simulink model "motion_joints"  (R2020a)
settings: Solver=ode1  StartTime=0.0  StopTime=10  FixedStep=0.001  RelTol=1e-3
libraries: robotcorelib x2, robotmaniplib x2
settings Model: Creator=Robot  LastModifiedBy=Robot

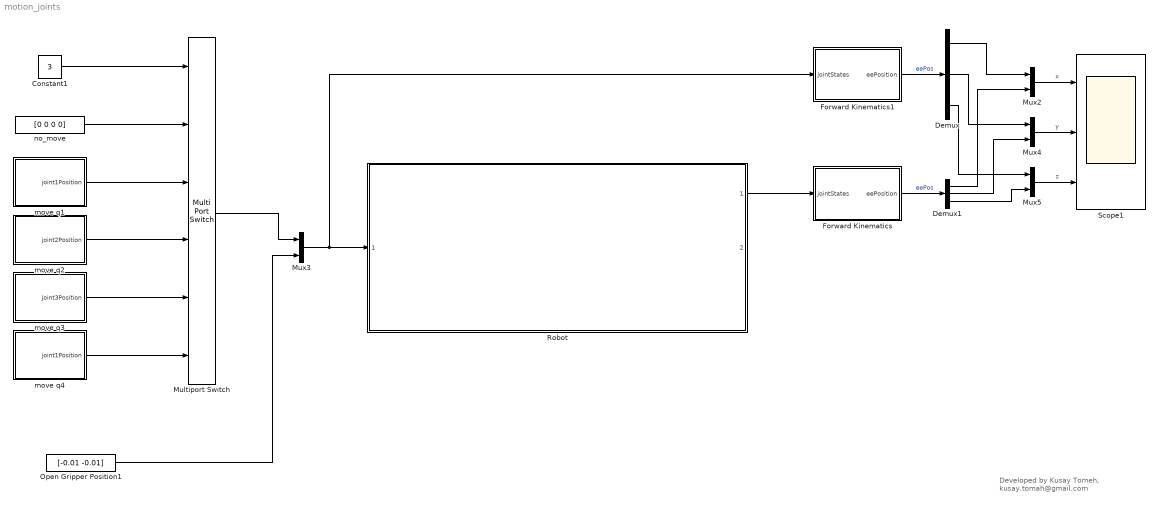
== system motion_joints ==
  note: Developed by Kusay Tomeh,
      | kusay.tomah@gmail.com
  Constant1 : Constant  Value=3
  Demux : Demux  Outputs=3
  Demux1 : Demux  Outputs=3
  Forward Kinematics : Subsystem
  Forward Kinematics1 : Subsystem
  Multiport Switch : MultiPortSwitch  Inputs=5
  Mux{2..5} (4 alike) : Mux  Inputs=2
  Open Gripper Position1 : Constant  Value=[-0.01 -0.01]
  Robot : Subsystem  ReferencedSubsystem=RobotModelWithFloor
  Scope1 : Scope  NumInputPorts=3
  move q1 : Subsystem
  move q2 : Subsystem
  move q3 : Subsystem
  move q4 : Subsystem
  no_move : Constant  Value=[0 0 0 0]
  wires:
  Mux3/1 -> Forward Kinematics1/1(jointStates), Robot/1
  Open Gripper Position1/1 -> Mux3/2
  move q4/1(joint1Position) -> Multiport Switch/6
  move q3/1(joint3Position) -> Multiport Switch/5
  move q2/1(joint2Position) -> Multiport Switch/4
  move q1/1(joint1Position) -> Multiport Switch/3
  Constant1/1 -> Multiport Switch/1
  Mux2/1 -> Scope1/1  "x"
  Multiport Switch/1 -> Mux3/1
  Demux1/2 -> Mux4/2
  Mux4/1 -> Scope1/2  "y"
  Demux/1 -> Mux2/1
  Demux/3 -> Mux5/1
  Demux1/3 -> Mux5/2
  Robot/1 -> Forward Kinematics/1(jointStates)
  Demux/2 -> Mux4/1
  Mux5/1 -> Scope1/3  "z"
  Demux1/1 -> Mux2/2
  Forward Kinematics/1(eePosition) -> Demux1/1  "eePos"
  Forward Kinematics1/1(eePosition) -> Demux/1  "eePos"
  no_move/1 -> Multiport Switch/2

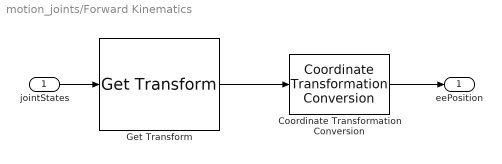
== system motion_joints/Forward Kinematics ==
  jointStates : Inport
  Coordinate Transformation Conversion : robotcorelib/Coordinate Transformation Conversion  InputRepresentation=Homogeneous Transformation  InputEulerSequence=ZYX  ShowTrVecInputPort=on  OutputRepresentation=Translation Vector  OutputEulerSequence=ZYX  ShowTrVecOutputPort=on  SimulateUsing=Code generation
      settings: SourceProductBaseCode=NV,RO,RR
      settings: AttributesFormatString=|
      | %<InputRepresentation>
      | to %<OutputRepresentation>
  Get Transform : robotmaniplib/Get Transform  RigidBodyTree=robot  SourceBody=end_effector  TargetBody=world  SimulateUsing=Interpreted execution
  eePosition : Outport  VectorParamsAs1DForOutWhenUnconnected=off
  wires:
  jointStates/1 -> Get Transform/1
  Coordinate Transformation Conversion/1 -> eePosition/1
  Get Transform/1 -> Coordinate Transformation Conversion/1

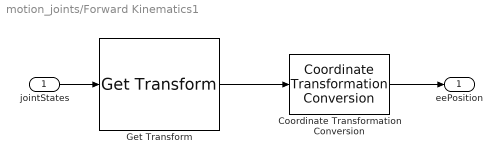
== system motion_joints/Forward Kinematics1 ==
  jointStates : Inport
  Coordinate Transformation Conversion : robotcorelib/Coordinate Transformation Conversion  InputRepresentation=Homogeneous Transformation  InputEulerSequence=ZYX  ShowTrVecInputPort=on  OutputRepresentation=Translation Vector  OutputEulerSequence=ZYX  ShowTrVecOutputPort=on  SimulateUsing=Code generation
      settings: SourceProductBaseCode=NV,RO,RR
      settings: AttributesFormatString=|
      | %<InputRepresentation>
      | to %<OutputRepresentation>
  Get Transform : robotmaniplib/Get Transform  RigidBodyTree=robot  SourceBody=end_effector  TargetBody=world  SimulateUsing=Interpreted execution
  eePosition : Outport  VectorParamsAs1DForOutWhenUnconnected=off
  wires:
  Get Transform/1 -> Coordinate Transformation Conversion/1
  Coordinate Transformation Conversion/1 -> eePosition/1
  jointStates/1 -> Get Transform/1

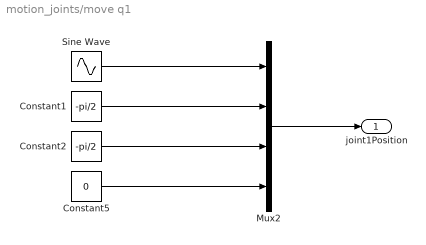
== system motion_joints/move q1 ==
  Constant1 : Constant  Value=-pi/2
  Constant2 : Constant  Value=-pi/2
  Constant5 : Constant  Value=0
  Mux2 : Mux
  Sine Wave : Sin  Amplitude=3.14  SampleTime=0
  joint1Position : Outport
  wires:
  Constant5/1 -> Mux2/4
  Constant2/1 -> Mux2/3
  Mux2/1 -> joint1Position/1
  Sine Wave/1 -> Mux2/1
  Constant1/1 -> Mux2/2

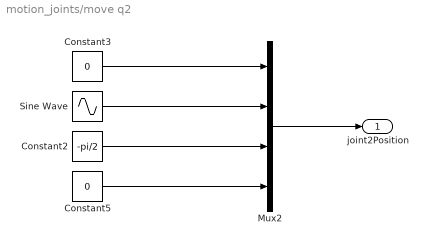
== system motion_joints/move q2 ==
  Constant2 : Constant  Value=-pi/2
  Constant3 : Constant  Value=0
  Constant5 : Constant  Value=0
  Mux2 : Mux
  Sine Wave : Sin  Amplitude=pi/2  SampleTime=0
  joint2Position : Outport
  wires:
  Sine Wave/1 -> Mux2/2
  Constant3/1 -> Mux2/1
  Mux2/1 -> joint2Position/1
  Constant2/1 -> Mux2/3
  Constant5/1 -> Mux2/4

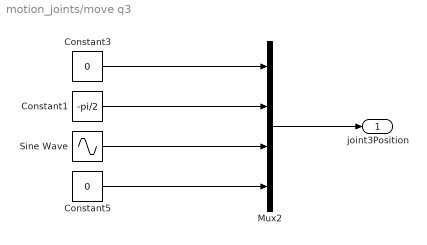
== system motion_joints/move q3 ==
  Constant1 : Constant  Value=-pi/2
  Constant3 : Constant  Value=0
  Constant5 : Constant  Value=0
  Mux2 : Mux
  Sine Wave : Sin  Amplitude=pi/3  SampleTime=0
  joint3Position : Outport
  wires:
  Constant5/1 -> Mux2/4
  Sine Wave/1 -> Mux2/3
  Mux2/1 -> joint3Position/1
  Constant1/1 -> Mux2/2
  Constant3/1 -> Mux2/1

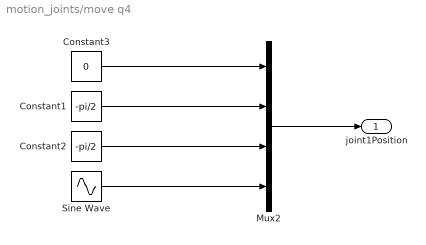
== system motion_joints/move q4 ==
  Constant1 : Constant  Value=-pi/2
  Constant2 : Constant  Value=-pi/2
  Constant3 : Constant  Value=0
  Mux2 : Mux
  Sine Wave : Sin  Amplitude=pi/2  SampleTime=0
  joint1Position : Outport
  wires:
  Constant1/1 -> Mux2/2
  Constant3/1 -> Mux2/1
  Mux2/1 -> joint1Position/1
  Constant2/1 -> Mux2/3
  Sine Wave/1 -> Mux2/4
